simulink model "LQR_lateral"  (R2016b)
settings: Solver=VariableStepAuto  StartTime=0.0  StopTime=20  RelTol=1e-3
undefined symbols (not defined in the file or in its folder): A_lat, B_lat, C_lat, D_lat, K_lat
libraries: dspsrcs4 x4
settings Model: Creator=yashm  LastModifiedBy=yashm

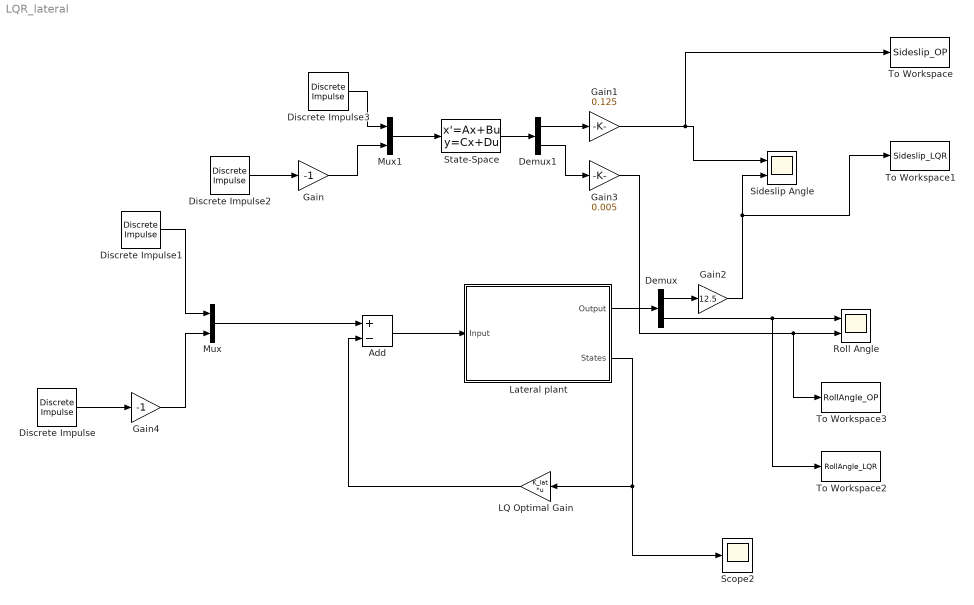
== system LQR_lateral ==
  Add : Sum  Inputs=+-
  Demux : Demux  Outputs=2
  Demux1 : Demux  Outputs=2
  Discrete Impulse{,1..3} (4 alike) : dspsrcs4/Discrete  Impulse  Delay=0  SampleTime=1  FrameSample=1  OutputFrames=off  dataType=double  isSigned=on  wordLen=16  udDataType=sfix(16)  fracBitsMode=Best precision  numFracBits=15  OutDataTypeStr=double  LastOutDataTypeStr=double
  Gain : Gain  Gain=-1
  Gain1 : Gain  Gain=0.125
  Gain2 : Gain  Gain=12.5
  Gain3 : Gain  Gain=0.005
  Gain4 : Gain  Gain=-1
  LQ Optimal Gain : Gain  Gain=K_lat  Multiplication=Matrix(K*u)
  "Lateral plant " : Subsystem
  Mux : Mux  Inputs=2
  Mux1 : Mux  Inputs=2
  "Roll Angle " : Scope  NumInputPorts=2
  Scope2 : Scope
  Sideslip Angle : Scope  NumInputPorts=2
  State-Space : StateSpace  A=A_lat  B=B_lat  C=C_lat  D=D_lat  X0=0
  To Workspace : ToWorkspace  VariableName=Sideslip_OP  SampleTime=0.001
      settings: Save2DSignal=2-D array (concatenate along first dimension)
  To Workspace1 : ToWorkspace  VariableName=Sideslip_LQR  SampleTime=0.001
      settings: Save2DSignal=2-D array (concatenate along first dimension)
  To Workspace2 : ToWorkspace  VariableName=RollAngle_LQR  SampleTime=0.001
      settings: Save2DSignal=2-D array (concatenate along first dimension)
  To Workspace3 : ToWorkspace  VariableName=RollAngle_OP  SampleTime=0.001
      settings: Save2DSignal=2-D array (concatenate along first dimension)
  wires:
  Demux/2 -> To Workspace2/1, "Roll Angle "/1
  Discrete Impulse1/1 -> Mux/1
  "Lateral plant "/1(Output) -> Demux/1
  Add/1 -> "Lateral plant "/1(Input)
  LQ Optimal Gain/1 -> Add/2
  Mux/1 -> Add/1
  "Lateral plant "/2(States) -> Scope2/1, LQ Optimal Gain/1
  State-Space/1 -> Demux1/1
  Mux1/1 -> State-Space/1
  Discrete Impulse3/1 -> Mux1/1
  Demux1/1 -> Gain1/1
  Gain1/1 -> To Workspace/1, Sideslip Angle/1
  Demux/1 -> Gain2/1
  Gain2/1 -> To Workspace1/1, Sideslip Angle/2
  Demux1/2 -> Gain3/1
  Gain3/1 -> To Workspace3/1, "Roll Angle "/2
  Discrete Impulse2/1 -> Gain/1
  Gain/1 -> Mux1/2
  Discrete Impulse/1 -> Gain4/1
  Gain4/1 -> Mux/2

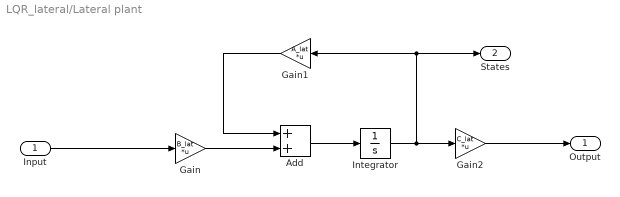
== system LQR_lateral/Lateral plant  ==
  Input : Inport
  Add : Sum
  Gain : Gain  Gain=B_lat  Multiplication=Matrix(K*u)
  Gain1 : Gain  Gain=A_lat  Multiplication=Matrix(K*u)
  Gain2 : Gain  Gain=C_lat  Multiplication=Matrix(K*u)
  Integrator : Integrator
  Output : Outport
  States : Outport  Port=2
  wires:
  Input/1 -> Gain/1
  Integrator/1 -> States/1, Gain1/1, Gain2/1
  Gain/1 -> Add/2
  Gain1/1 -> Add/1
  Gain2/1 -> Output/1
  Add/1 -> Integrator/1
